simulink model "Lab1_2"  (Simulink 8.0)
settings: Solver=ode3  StartTime=0.0  StopTime=10.0  FixedStep=0.001  RelTol=1e-3
undefined symbols (not defined in the file or in its folder): MultiQ, PCI, Quanser
libraries: rtwinlib x3
settings Model: Creator=Mehatronicki Sustavi  LastModifiedBy=Niko  SimulationMode=external  ExtModeTrigDuration=1000000
settings DataIOCC: SignalLoggingSaveFormat=ModelDataLogs
settings DebuggingCC: FcnCallInpInsideContextMsg=UseLocalSettings  StrictBusMsg=Warning
settings HardwareCC: ProdIntDivRoundTo=Zero  ProdEndianess=LittleEndian  ProdHWDeviceType=Generic->32-bit x86 compatible
settings RTWCC: SystemTargetFile=rtwin.tlc  TemplateMakefile=rtwin.tmf  Description=Real-Time Windows Target  ProcessScript=rtwin_make_rtw_hook  RTWCompilerOptimization=On
settings CodeAppCC: MaxIdLength=95
settings RTWinTargetCC: TargetLibSuffix=_rtwin.lib  TargetPreCompLibLocation=G:\Program Files\MATLAB\R2012b\toolbox\rtw\targets\rtwin\lib\win64  CodeReplacementLibrary=ANSI_C  RTWinDir=G:/Program Files/MATLAB/R2012b/toolbox/rtw/targets/rtwin  TargetArch=win64

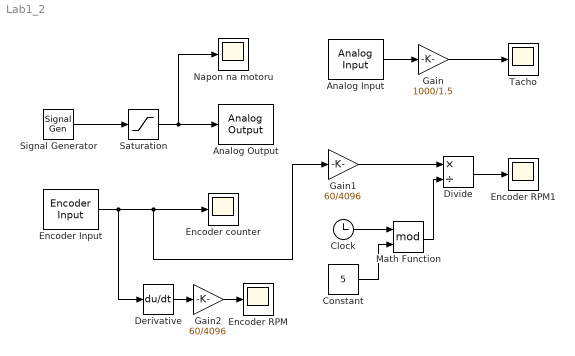
== system Lab1_2 ==
  Analog Input : rtwinlib/Analog Input  SampleTime=0.001  MaxMissedTicks=10  ShowMissedTicks=off  YieldWhenWaiting=off  DrvName=Quanser/MultiQ-PCI  DrvAddress=4294967295  DrvOptions=zeros(1,0)  Channels=2  RangeMode=1  VoltRange=1  DataType=1
      settings: AttributesFormatString=Quanser\nMultiQ-PCI [auto]
  Analog Output : rtwinlib/Analog Output  SampleTime=0.001  MaxMissedTicks=10  ShowMissedTicks=off  YieldWhenWaiting=off  DrvName=Quanser/MultiQ-PCI  DrvAddress=4294967295  DrvOptions=zeros(1,0)  Channels=1  RangeMode=1  VoltRange=1  InitialValue=0  FinalValue=0
      settings: AttributesFormatString=Quanser\nMultiQ-PCI [auto]
  Clock : Clock
  Constant : Constant  Value=5
  Derivative : Derivative  CoefficientInTFapproximation=0.0001
  Divide : Product  Inputs=*/
  Encoder Input : rtwinlib/Encoder Input  SampleTime=0.001  MaxMissedTicks=10  ShowMissedTicks=off  YieldWhenWaiting=off  DrvName=Quanser/MultiQ-PCI  DrvAddress=4294967295  DrvOptions=zeros(1,0)  Channels=1  QuadMode=3  IndexPulse=2  InputFilter=Inf  DataType=1
      settings: AttributesFormatString=Quanser\nMultiQ-PCI [auto]
  Encoder RPM : Scope
      settings: YMin=-5000  YMax=5000  SaveName=EncoderRPM
  Encoder RPM1 : Scope
      settings: YMin=-5000  YMax=5000  SaveName=EncoderRPM1
  Encoder counter : Scope
      settings: YMin=0  YMax=12000  SaveName=EncoderCnt
  Gain : Gain  Gain=1000/1.5
  Gain1 : Gain  Gain=60/4096
  Gain2 : Gain  Gain=60/4096
  Math Function : Math  Operator=mod  SaturateOnIntegerOverflow=on
  Napon na motoru : Scope
      settings: SaveName=NaponMotor
  Saturation : Saturate  UpperLimit=6  LowerLimit=-6
  Signal Generator : SignalGenerator  WaveForm=square  Amplitude=3  Frequency=0.1
  Tacho : Scope
      settings: YMin=-3500  YMax=3500  SaveName=Tacho
  wires:
  Signal Generator/1 -> Saturation/1
  Saturation/1 -> Analog Output/1, Napon na motoru/1
  Analog Input/1 -> Gain/1
  Gain/1 -> Tacho/1
  Encoder Input/1 -> Derivative/1, Encoder counter/1, Gain1/1
  Clock/1 -> Math Function/1
  Constant/1 -> Math Function/2
  Gain1/1 -> Divide/1
  Math Function/1 -> Divide/2
  Divide/1 -> Encoder RPM1/1
  Gain2/1 -> Encoder RPM/1
  Derivative/1 -> Gain2/1
